simulink model "SF049A_LoaMgr"  (R2013b)
settings: Solver=FixedStepDiscrete  SolverMode=SingleTasking  StartTime=0.0  StopTime=1  FixedStep=0.002  RelTol=1e-3
values from neighbouring files (symbols this model uses):
  CURRMEASLOAMTGTNMASK_CNT_U08 = DataDict.Constant    [SF049A_LoaMgr_DataDict.m]
  IVTRLOAMTGTNMASK_CNT_U08 = DataDict.Constant    [SF049A_LoaMgr_DataDict.m]
  LOAMAXSLEW_ULSPERSEC_F32 = DataDict.Constant    [SF049A_LoaMgr_DataDict.m]
  LoaMgrCurrIvtrMtgtnRate = DataDict.Calibration    [SF049A_LoaMgr_DataDict.m]
  LoaMgrCurrIvtrMtgtnSca = DataDict.Calibration    [SF049A_LoaMgr_DataDict.m]
  LoaMgrCurrIvtrMtgtnScaZeroEna = DataDict.Calibration    [SF049A_LoaMgr_DataDict.m]
  LoaMgrCurrMeasIdptSig0Resp = DataDict.Calibration    [SF049A_LoaMgr_DataDict.m]
  LoaMgrCurrMeasIdptSig1Resp = DataDict.Calibration    [SF049A_LoaMgr_DataDict.m]
  LoaMgrCurrMeasIdptSig2Resp = DataDict.Calibration    [SF049A_LoaMgr_DataDict.m]
  LoaMgrCurrMeasIdptSigFltThd = DataDict.Calibration    [SF049A_LoaMgr_DataDict.m]
  LoaMgrCurrMeasMtgtnRate = DataDict.Calibration    [SF049A_LoaMgr_DataDict.m]
  LoaMgrCurrMeasMtgtnSca = DataDict.Calibration    [SF049A_LoaMgr_DataDict.m]
  LoaMgrCurrMeasMtgtnScaZeroEna = DataDict.Calibration    [SF049A_LoaMgr_DataDict.m]
  LoaMgrFadeOutStRate = DataDict.Calibration    [SF049A_LoaMgr_DataDict.m]
  LoaMgrHwTqIdptSig0NoTqLoaResp = DataDict.Calibration    [SF049A_LoaMgr_DataDict.m]
  LoaMgrHwTqIdptSig1NoTqLoaResp = DataDict.Calibration    [SF049A_LoaMgr_DataDict.m]
  LoaMgrHwTqIdptSig2Resp = DataDict.Calibration    [SF049A_LoaMgr_DataDict.m]
  LoaMgrHwTqIdptSig4Resp = DataDict.Calibration    [SF049A_LoaMgr_DataDict.m]
  LoaMgrHwTqIdptSigFltThd = DataDict.Calibration    [SF049A_LoaMgr_DataDict.m]
  LoaMgrHwTqLoaAvlResp = DataDict.Calibration    [SF049A_LoaMgr_DataDict.m]
  LoaMgrIvtrIdptSig0Resp = DataDict.Calibration    [SF049A_LoaMgr_DataDict.m]
  LoaMgrIvtrIdptSig1Resp = DataDict.Calibration    [SF049A_LoaMgr_DataDict.m]
  LoaMgrIvtrIdptSig2Resp = DataDict.Calibration    [SF049A_LoaMgr_DataDict.m]
  LoaMgrIvtrIdptSigFltThd = DataDict.Calibration    [SF049A_LoaMgr_DataDict.m]
  LoaMgrIvtrMtgtnRate = DataDict.Calibration    [SF049A_LoaMgr_DataDict.m]
  LoaMgrIvtrMtgtnSca = DataDict.Calibration    [SF049A_LoaMgr_DataDict.m]
  LoaMgrIvtrMtgtnScaZeroEna = DataDict.Calibration    [SF049A_LoaMgr_DataDict.m]
  LoaMgrLimdStRate = DataDict.Calibration    [SF049A_LoaMgr_DataDict.m]
  LoaMgrLimdStSca = DataDict.Calibration    [SF049A_LoaMgr_DataDict.m]
  LoaMgrMotAgAvlSnsrlsResp = DataDict.Calibration    [SF049A_LoaMgr_DataDict.m]
  LoaMgrMotAgIdptSig0NoSnsrlsResp = DataDict.Calibration    [SF049A_LoaMgr_DataDict.m]
  LoaMgrMotAgIdptSig1NoSnsrlsResp = DataDict.Calibration    [SF049A_LoaMgr_DataDict.m]
  LoaMgrMotAgIdptSig2Resp = DataDict.Calibration    [SF049A_LoaMgr_DataDict.m]
  LoaMgrMotAgIdptSig3Resp = DataDict.Calibration    [SF049A_LoaMgr_DataDict.m]
  LoaMgrMotAgIdptSigFltThd = DataDict.Calibration    [SF049A_LoaMgr_DataDict.m]
  LoaMgrMotAgMtgtnRate = DataDict.Calibration    [SF049A_LoaMgr_DataDict.m]
  LoaMgrMotAgMtgtnSca = DataDict.Calibration    [SF049A_LoaMgr_DataDict.m]
  LoaMgrMotAgMtgtnScaZeroEna = DataDict.Calibration    [SF049A_LoaMgr_DataDict.m]
  LOASCAONE_ULS_F32 = DataDict.Constant    [SF049A_LoaMgr_DataDict.m]
  LOASCAZERO_ULS_F32 = DataDict.Constant    [SF049A_LoaMgr_DataDict.m]
  LOASTIMDTSHTDWN_CNT_U08 = DataDict.Constant    [SF049A_LoaMgr_DataDict.m]
  LOASTNORM_CNT_U08 = DataDict.Constant    [SF049A_LoaMgr_DataDict.m]
  LOASTSWMTGTN_CNT_U08 = DataDict.Constant    [SF049A_LoaMgr_DataDict.m]
  MAXCURRMEASIDPTSIGALLWD_CNT_U08 = DataDict.Constant    [SF049A_LoaMgr_DataDict.m]
  MAXHWTQIDPTSIGALLWD_CNT_U08 = DataDict.Constant    [SF049A_LoaMgr_DataDict.m]
  MAXIVTRIDPTSIGALLWD_CNT_U08 = DataDict.Constant    [SF049A_LoaMgr_DataDict.m]
  MAXMOTAGMECLIDPTSIGALLWD_CNT_U08 = DataDict.Constant    [SF049A_LoaMgr_DataDict.m]
  NODEBSTEP_CNT_U16 = DataDict.Constant    [SF049A_LoaMgr_DataDict.m]
undefined symbols (not defined in the file or in its folder): LoaSt1, NtcNr1, NtcSts1, SigQlfr1
libraries: simulink x43, NxtrMin x4, NxtrMax x4, NxtrLim x2
(part 4 of 8)

== system SF049A_LoaMgr/LoaMgr/LoaMgrPer1/Arbitrate_Responses/SelFinalResp ==
  note: Pick the most severe of all the requested responses.
      |
      | 5 Immediate Shutdown  (most severe)
      | 4 Controlled Shutdown
      | 3 FadeOut
      | 2 Software-based Mitigation
      | 1 Reduced Performance
      | 0 Normal Operation       (least severe)
  MultiMtgtnResp : Inport  RequirementInfo="{'linktype_rmi_doors' '0000bab3 (/E-STEER Core/SubSystem Specifications/Application Functions/SF049A Loss of Assist Manager)' '#SF049A_84' 'true' 'REQ:  SF049A_84' '' } %GIDa_54734b91_5608_48ea_8068_35ba43353152"
  HwTqResp : Inport  RequirementInfo="{'linktype_rmi_doors' '0000bab3 (/E-STEER Core/SubSystem Specifications/Application Functions/SF049A Loss of Assist Manager)' '#SF049A_84' 'true' 'REQ:  SF049A_84' '' } %GIDa_c3761ef3_9e8d_4836_b42a_0c95799c1a90"  Port=2
  MotAgResp : Inport  RequirementInfo="{'linktype_rmi_doors' '0000bab3 (/E-STEER Core/SubSystem Specifications/Application Functions/SF049A Loss of Assist Manager)' '#SF049A_84' 'true' 'REQ:  SF049A_84' '' } %GIDa_49dd4887_96d7_4bb8_87d7_95367e2f50fb"  Port=3
  CurrMeasResp : Inport  RequirementInfo="{'linktype_rmi_doors' '0000bab3 (/E-STEER Core/SubSystem Specifications/Application Functions/SF049A Loss of Assist Manager)' '#SF049A_84' 'true' 'REQ:  SF049A_84' '' } %GIDa_84bf3833_e209_43be_a485_a63c89bdf184"  Port=4
  IvtrResp : Inport  RequirementInfo="{'linktype_rmi_doors' '0000bab3 (/E-STEER Core/SubSystem Specifications/Application Functions/SF049A Loss of Assist Manager)' '#SF049A_84' 'true' 'REQ:  SF049A_84' '' } %GIDa_dd1bf10a_41ed_4001_b74c_b927cf7e28c7"  Port=5
  CopyRight2 : Subsystem  Description=|  mask(Copyright Information){none=on}
      | Copyright info block.                                               
      |                                                                     
      | Place copyright information at the top of every subsystem in design.
      mask prompts: none "No parameters"
      mask help: Place copyright information at the top of every subsystem in design.
      mask Display:
      | NxtrConf = 'Nexteer Confidential';
      | 
      | sys = bdroot; %handle for the current model ("system")
      | first = get_param(sys,'Created');
      | first = first(end-3:end);  %year is last four digits
      | 
      | last = get_param(sys,'LastModifiedDate');
      | if isempty(last)
      |     last = datestr(now,'yyyy');
      | else
      |     last = last(end-3:end);
      | end
      | 
      | if strcmp(first,last)
      |     fprintf('%s -- Copyright %s Nexteer',NxtrConf,first)
      | else
      |     fprintf('%s -- %s%s- %s Nexteer',NxtrConf,char(169),first,last)
      | end
  F1 : Subsystem  RequirementInfo="{'linktype_rmi_doors' '0000bab3 (/E-STEER Core/SubSystem Specifications/Application Functions/SF049A Loss of Assist Manager)' '#SF049A_84' 'true' 'REQ:  SF049A_84' '' } %GIDa_43cd8944_2563_4272_8a81_50c14054d8ba"  TreatAsAtomicUnit=on
      settings: RTWSystemCode=Inline
  F2 : Subsystem  RequirementInfo="{'linktype_rmi_doors' '0000bab3 (/E-STEER Core/SubSystem Specifications/Application Functions/SF049A Loss of Assist Manager)' '#SF049A_84' 'true' 'REQ:  SF049A_84' '' } %GIDa_ad4154bc_5125_4599_b026_eafd9bdc2db0"  TreatAsAtomicUnit=on
      settings: RTWSystemCode=Inline
  Fade_Out : Subsystem  RequirementInfo="{'linktype_rmi_doors' '0000bab3 (/E-STEER Core/SubSystem Specifications/Application Functions/SF049A Loss of Assist Manager)' '#SF049A_84' 'true' 'REQ:  SF049A_84' '' } %GIDa_e73d73a9_eff4_41e2_9d30_bb96570f7ea9"  TreatAsAtomicUnit=on
      settings: RTWSystemCode=Inline
  Fade_Out1 : Subsystem  RequirementInfo="{'linktype_rmi_doors' '0000bab3 (/E-STEER Core/SubSystem Specifications/Application Functions/SF049A Loss of Assist Manager)' '#SF049A_84' 'true' 'REQ:  SF049A_84' '' } %GIDa_df16c958_8064_4140_9dc4_1de426c4fa71"  TreatAsAtomicUnit=on
      settings: RTWSystemCode=Inline
  Merge : Merge  RequirementInfo="{'linktype_rmi_doors' '0000bab3 (/E-STEER Core/SubSystem Specifications/Application Functions/SF049A Loss of Assist Manager)' '#SF049A_84' 'true' 'REQ:  SF049A_84' '' } %GIDa_bf53b07b_d7b9_4c96_87f9_e1354b1860d8"  Inputs=7
  MinMax : MinMax  RequirementInfo="{'linktype_rmi_doors' '0000bab3 (/E-STEER Core/SubSystem Specifications/Application Functions/SF049A Loss of Assist Manager)' '#SF049A_84' 'true' 'REQ:  SF049A_84' '' } %GIDa_e56cb4a9_e669_420e_96d1_e3295adf3ac5"  Function=max  Inputs=5
  Norm : Subsystem  RequirementInfo="{'linktype_rmi_doors' '0000bab3 (/E-STEER Core/SubSystem Specifications/Application Functions/SF049A Loss of Assist Manager)' '#SF049A_84' 'true' 'REQ:  SF049A_84' '' } %GIDa_79fd85a7_d991_4c90_8f93_f8588bbab999"  TreatAsAtomicUnit=on
      settings: RTWSystemCode=Inline
  Reduced : Subsystem  RequirementInfo="{'linktype_rmi_doors' '0000bab3 (/E-STEER Core/SubSystem Specifications/Application Functions/SF049A Loss of Assist Manager)' '#SF049A_84' 'true' 'REQ:  SF049A_84' '' } %GIDa_282ff44a_ee82_477d_994c_5b522cb9007f"  TreatAsAtomicUnit=on
      settings: RTWSystemCode=Inline
  SwBasd_Mtgtn : Subsystem  RequirementInfo="{'linktype_rmi_doors' '0000bab3 (/E-STEER Core/SubSystem Specifications/Application Functions/SF049A Loss of Assist Manager)' '#SF049A_84' 'true' 'REQ:  SF049A_84' '' } %GIDa_b7021016_4e5a_41fb_b8b0_41c73dc15fee"  TreatAsAtomicUnit=on
      settings: RTWSystemCode=Inline
  Switch Case : SwitchCase  RequirementInfo="{'linktype_rmi_doors' '0000bab3 (/E-STEER Core/SubSystem Specifications/Application Functions/SF049A Loss of Assist Manager)' '#SF049A_84' 'true' 'REQ:  SF049A_84' '' } %GIDa_44be8c31_fd6f_47a2_aa3d_457bbc5e3cf2"  CaseConditions={5,4,3,2,1,0}
  LoaSt : Outport  RequirementInfo="{'linktype_rmi_doors' '0000bab3 (/E-STEER Core/SubSystem Specifications/Application Functions/SF049A Loss of Assist Manager)' '#SF049A_84' 'true' 'REQ:  SF049A_84' '' } %GIDa_2917bb2b_4bd4_4079_ac09_4ef15e442a03"
  wires:
  SwBasd_Mtgtn/1(LoaSt) -> Merge/4
  Switch Case/7 -> Fade_Out1/Action
  MultiMtgtnResp/1 -> MinMax/1
  Fade_Out1/1(LoaSt) -> Merge/7
  Switch Case/6 -> Norm/Action
  Norm/1(LoaSt) -> Merge/6
  MinMax/1 -> Switch Case/1
  Switch Case/1 -> F1/Action
  F2/1(LoaSt) -> Merge/2
  Merge/1 -> LoaSt/1
  Fade_Out/1(LoaSt) -> Merge/3
  Switch Case/5 -> Reduced/Action
  Switch Case/3 -> Fade_Out/Action
  IvtrResp/1 -> MinMax/5
  Reduced/1(LoaSt) -> Merge/5
  Switch Case/2 -> F2/Action
  CurrMeasResp/1 -> MinMax/4
  F1/1(LoaSt) -> Merge/1
  HwTqResp/1 -> MinMax/2
  MotAgResp/1 -> MinMax/3
  Switch Case/4 -> SwBasd_Mtgtn/Action

== system SF049A_LoaMgr/LoaMgr/LoaMgrPer1/Assign_Scale/CopyRight2 ==

== system SF049A_LoaMgr/LoaMgr/LoaMgrPer1/Assign_Scale/F1 ==
  F1 : ActionPort  ActionType=else
  Constant1 : Constant  Value=LOASCAZERO_ULS_F32
  Constant2 : Constant  Value=LOAMAXSLEW_ULSPERSEC_F32
  CopyRight2 : Subsystem  Description=|  mask(Copyright Information){none=on}
      | Copyright info block.                                               
      |                                                                     
      | Place copyright information at the top of every subsystem in design.
      mask prompts: none "No parameters"
      mask help: Place copyright information at the top of every subsystem in design.
      mask Display:
      | NxtrConf = 'Nexteer Confidential';
      | 
      | sys = bdroot; %handle for the current model ("system")
      | first = get_param(sys,'Created');
      | first = first(end-3:end);  %year is last four digits
      | 
      | last = get_param(sys,'LastModifiedDate');
      | if isempty(last)
      |     last = datestr(now,'yyyy');
      | else
      |     last = last(end-3:end);
      | end
      | 
      | if strcmp(first,last)
      |     fprintf('%s -- Copyright %s Nexteer',NxtrConf,first)
      | else
      |     fprintf('%s -- %s%s- %s Nexteer',NxtrConf,char(169),first,last)
      | end
  Sca : Outport
  Rate : Outport  Port=2
  wires:
  Constant1/1 -> Sca/1
  Constant2/1 -> Rate/1

== system SF049A_LoaMgr/LoaMgr/LoaMgrPer1/Assign_Scale/F2 ==
  F2 : ActionPort  ActionType=elseif
  Constant1 : Constant  Value=LOASCAZERO_ULS_F32
  Constant2 : Constant  Value=LOAMAXSLEW_ULSPERSEC_F32
  CopyRight2 : Subsystem  Description=|  mask(Copyright Information){none=on}
      | Copyright info block.                                               
      |                                                                     
      | Place copyright information at the top of every subsystem in design.
      mask prompts: none "No parameters"
      mask help: Place copyright information at the top of every subsystem in design.
      mask Display:
      | NxtrConf = 'Nexteer Confidential';
      | 
      | sys = bdroot; %handle for the current model ("system")
      | first = get_param(sys,'Created');
      | first = first(end-3:end);  %year is last four digits
      | 
      | last = get_param(sys,'LastModifiedDate');
      | if isempty(last)
      |     last = datestr(now,'yyyy');
      | else
      |     last = last(end-3:end);
      | end
      | 
      | if strcmp(first,last)
      |     fprintf('%s -- Copyright %s Nexteer',NxtrConf,first)
      | else
      |     fprintf('%s -- %s%s- %s Nexteer',NxtrConf,char(169),first,last)
      | end
  Sca : Outport
  Rate : Outport  Port=2
  wires:
  Constant1/1 -> Sca/1
  Constant2/1 -> Rate/1

== system SF049A_LoaMgr/LoaMgr/LoaMgrPer1/Assign_Scale/Fade ==
  Fade : ActionPort  ActionType=elseif
  Constant1 : Constant  Value=LOASCAZERO_ULS_F32
  Constant2 : Constant  Value=LoaMgrFadeOutStRate
  CopyRight2 : Subsystem  Description=|  mask(Copyright Information){none=on}
      | Copyright info block.                                               
      |                                                                     
      | Place copyright information at the top of every subsystem in design.
      mask prompts: none "No parameters"
      mask help: Place copyright information at the top of every subsystem in design.
      mask Display:
      | NxtrConf = 'Nexteer Confidential';
      | 
      | sys = bdroot; %handle for the current model ("system")
      | first = get_param(sys,'Created');
      | first = first(end-3:end);  %year is last four digits
      | 
      | last = get_param(sys,'LastModifiedDate');
      | if isempty(last)
      |     last = datestr(now,'yyyy');
      | else
      |     last = last(end-3:end);
      | end
      | 
      | if strcmp(first,last)
      |     fprintf('%s -- Copyright %s Nexteer',NxtrConf,first)
      | else
      |     fprintf('%s -- %s%s- %s Nexteer',NxtrConf,char(169),first,last)
      | end
  Sca : Outport
  Rate : Outport  Port=2
  wires:
  Constant1/1 -> Sca/1
  Constant2/1 -> Rate/1

== system SF049A_LoaMgr/LoaMgr/LoaMgrPer1/Assign_Scale/Limd ==
  Reduced : ActionPort  ActionType=elseif
  Constant1 : Constant  Value=LoaMgrLimdStSca
  Constant2 : Constant  Value=LoaMgrLimdStRate
  CopyRight2 : Subsystem  Description=|  mask(Copyright Information){none=on}
      | Copyright info block.                                               
      |                                                                     
      | Place copyright information at the top of every subsystem in design.
      mask prompts: none "No parameters"
      mask help: Place copyright information at the top of every subsystem in design.
      mask Display:
      | NxtrConf = 'Nexteer Confidential';
      | 
      | sys = bdroot; %handle for the current model ("system")
      | first = get_param(sys,'Created');
      | first = first(end-3:end);  %year is last four digits
      | 
      | last = get_param(sys,'LastModifiedDate');
      | if isempty(last)
      |     last = datestr(now,'yyyy');
      | else
      |     last = last(end-3:end);
      | end
      | 
      | if strcmp(first,last)
      |     fprintf('%s -- Copyright %s Nexteer',NxtrConf,first)
      | else
      |     fprintf('%s -- %s%s- %s Nexteer',NxtrConf,char(169),first,last)
      | end
  Sca : Outport
  Rate : Outport  Port=2
  wires:
  Constant1/1 -> Sca/1
  Constant2/1 -> Rate/1

== system SF049A_LoaMgr/LoaMgr/LoaMgrPer1/Assign_Scale/Norm ==
  Normal : ActionPort  ActionType=then
  Constant1 : Constant  Value=LOASCAONE_ULS_F32
  Constant2 : Constant  Value=LOAMAXSLEW_ULSPERSEC_F32
  CopyRight2 : Subsystem  Description=|  mask(Copyright Information){none=on}
      | Copyright info block.                                               
      |                                                                     
      | Place copyright information at the top of every subsystem in design.
      mask prompts: none "No parameters"
      mask help: Place copyright information at the top of every subsystem in design.
      mask Display:
      | NxtrConf = 'Nexteer Confidential';
      | 
      | sys = bdroot; %handle for the current model ("system")
      | first = get_param(sys,'Created');
      | first = first(end-3:end);  %year is last four digits
      | 
      | last = get_param(sys,'LastModifiedDate');
      | if isempty(last)
      |     last = datestr(now,'yyyy');
      | else
      |     last = last(end-3:end);
      | end
      | 
      | if strcmp(first,last)
      |     fprintf('%s -- Copyright %s Nexteer',NxtrConf,first)
      | else
      |     fprintf('%s -- %s%s- %s Nexteer',NxtrConf,char(169),first,last)
      | end
  Sca : Outport
  Rate : Outport  Port=2
  wires:
  Constant1/1 -> Sca/1
  Constant2/1 -> Rate/1

== system SF049A_LoaMgr/LoaMgr/LoaMgrPer1/Assign_Scale/SwMtgtn ==
  SwMtgtnEn : Inport
  SwMtgtn : ActionPort  ActionType=elseif
  CopyRight2 : Subsystem  Description=|  mask(Copyright Information){none=on}
      | Copyright info block.                                               
      |                                                                     
      | Place copyright information at the top of every subsystem in design.
      mask prompts: none "No parameters"
      mask help: Place copyright information at the top of every subsystem in design.
      mask Display:
      | NxtrConf = 'Nexteer Confidential';
      | 
      | sys = bdroot; %handle for the current model ("system")
      | first = get_param(sys,'Created');
      | first = first(end-3:end);  %year is last four digits
      | 
      | last = get_param(sys,'LastModifiedDate');
      | if isempty(last)
      |     last = datestr(now,'yyyy');
      | else
      |     last = last(end-3:end);
      | end
      | 
      | if strcmp(first,last)
      |     fprintf('%s -- Copyright %s Nexteer',NxtrConf,first)
      | else
      |     fprintf('%s -- %s%s- %s Nexteer',NxtrConf,char(169),first,last)
      | end
  Data Store Read1 : DataStoreRead  Priority=1  DataStoreName=PrevVltgModSrc
  Data Store Read3 : DataStoreRead  Priority=1  DataStoreName=PrevMotAgLoaMtgtnEna
  Data Store Write1 : DataStoreWrite  Priority=2  DataStoreName=PrevVltgModSrc
  Data Store Write2 : DataStoreWrite  Priority=2  DataStoreName=PrevMotAgLoaMtgtnEna
  Demux : Demux
  HwTqTrue : Subsystem  RequirementInfo="{'linktype_rmi_doors' '0000bab3 (/E-STEER Core/SubSystem Specifications/Application Functions/SF049A Loss of Assist Manager)' '#SF049A_99' 'true' 'REQ:  SF049A_99' '' } %GIDa_7b14d0c5_f882_4af7_a11e_f83b181f5ec7"  TreatAsAtomicUnit=on
      settings: RTWSystemCode=Inline
  If : If  RequirementInfo="{'linktype_rmi_doors' '0000bab3 (/E-STEER Core/SubSystem Specifications/Application Functions/SF049A Loss of Assist Manager)' '#SF049A_99' 'true' 'REQ:  SF049A_99' '' ; 'linktype_rmi_doors' '0000bab3 (/E-STEER Core/SubSystem Specifications/Application Functions/SF049A Loss of Assist Manager)' '#SF049A_100' 'true' 'REQ:  SF049A_100' '' ; 'linktype_rmi_doors' '0000bab3 (/E-STEER Core/SubSystem Specifications/Application Functions/SF049A Loss of Assist Manager)' '#SF049A_107' 'true' 'REQ:  SF049A_107' '' ; 'linktype_rmi_doors' '0000bab3 (/E-STEER Core/SubSystem Specifications/Application Functions/SF049A Loss of Assist Manager)' '#SF049A_108' 'true' 'REQ:  SF049A_108' '' } %GIDa_e3d1a53d_44ce_4ebb_b524_70ede7db229d"  NumInputs=2  IfExpression=u1  ElseIfExpressions=u2
  MaskBooleans : Subsystem
  Merge : Merge  RequirementInfo="{'linktype_rmi_doors' '0000bab3 (/E-STEER Core/SubSystem Specifications/Application Functions/SF049A Loss of Assist Manager)' '#SF049A_99' 'true' 'REQ:  SF049A_99' '' ; 'linktype_rmi_doors' '0000bab3 (/E-STEER Core/SubSystem Specifications/Application Functions/SF049A Loss of Assist Manager)' '#SF049A_100' 'true' 'REQ:  SF049A_100' '' ; 'linktype_rmi_doors' '0000bab3 (/E-STEER Core/SubSystem Specifications/Application Functions/SF049A Loss of Assist Manager)' '#SF049A_107' 'true' 'REQ:  SF049A_107' '' ; 'linktype_rmi_doors' '0000bab3 (/E-STEER Core/SubSystem Specifications/Application Functions/SF049A Loss of Assist Manager)' '#SF049A_108' 'true' 'REQ:  SF049A_108' '' } %GIDa_35100d15_d4ea_4b72_b96f_d7a4004a9afa"  Inputs=3
  Merge1 : Merge  RequirementInfo="{'linktype_rmi_doors' '0000bab3 (/E-STEER Core/SubSystem Specifications/Application Functions/SF049A Loss of Assist Manager)' '#SF049A_99' 'true' 'REQ:  SF049A_99' '' ; 'linktype_rmi_doors' '0000bab3 (/E-STEER Core/SubSystem Specifications/Application Functions/SF049A Loss of Assist Manager)' '#SF049A_100' 'true' 'REQ:  SF049A_100' '' ; 'linktype_rmi_doors' '0000bab3 (/E-STEER Core/SubSystem Specifications/Application Functions/SF049A Loss of Assist Manager)' '#SF049A_107' 'true' 'REQ:  SF049A_107' '' ; 'linktype_rmi_doors' '0000bab3 (/E-STEER Core/SubSystem Specifications/Application Functions/SF049A Loss of Assist Manager)' '#SF049A_108' 'true' 'REQ:  SF049A_108' '' } %GIDa_747b6afd_1894_45a5_8818_39983e3267c2"  Inputs=3
  MotAgTrue : Subsystem  RequirementInfo="{'linktype_rmi_doors' '0000bab3 (/E-STEER Core/SubSystem Specifications/Application Functions/SF049A Loss of Assist Manager)' '#SF049A_100' 'true' 'REQ:  SF049A_100' '' } %GIDa_ffb79f06_004e_4cb8_9570_e4a0dcfed390"  TreatAsAtomicUnit=on
      settings: RTWSystemCode=Inline
  OthersTrue : Subsystem  RequirementInfo="{'linktype_rmi_doors' '0000bab3 (/E-STEER Core/SubSystem Specifications/Application Functions/SF049A Loss of Assist Manager)' '#SF049A_107' 'true' 'REQ:  SF049A_107' '' ; 'linktype_rmi_doors' '0000bab3 (/E-STEER Core/SubSystem Specifications/Application Functions/SF049A Loss of Assist Manager)' '#SF049A_108' 'true' 'REQ:  SF049A_108' '' } %GIDa_b6d2c039_d125_4c6d_9822_c6a7833ff1f7"  TreatAsAtomicUnit=on
      settings: RTWSystemCode=Inline
  Sca : Outport  RequirementInfo="{'linktype_rmi_doors' '0000bab3 (/E-STEER Core/SubSystem Specifications/Application Functions/SF049A Loss of Assist Manager)' '#SF049A_99' 'true' 'REQ:  SF049A_99' '' ; 'linktype_rmi_doors' '0000bab3 (/E-STEER Core/SubSystem Specifications/Application Functions/SF049A Loss of Assist Manager)' '#SF049A_100' 'true' 'REQ:  SF049A_100' '' ; 'linktype_rmi_doors' '0000bab3 (/E-STEER Core/SubSystem Specifications/Application Functions/SF049A Loss of Assist Manager)' '#SF049A_107' 'true' 'REQ:  SF049A_107' '' ; 'linktype_rmi_doors' '0000bab3 (/E-STEER Core/SubSystem Specifications/Application Functions/SF049A Loss of Assist Manager)' '#SF049A_108' 'true' 'REQ:  SF049A_108' '' } %GIDa_85f88b7e_b82d_4e96_8747_a438a2f288cc"
  Rate : Outport  RequirementInfo="{'linktype_rmi_doors' '0000bab3 (/E-STEER Core/SubSystem Specifications/Application Functions/SF049A Loss of Assist Manager)' '#SF049A_99' 'true' 'REQ:  SF049A_99' '' ; 'linktype_rmi_doors' '0000bab3 (/E-STEER Core/SubSystem Specifications/Application Functions/SF049A Loss of Assist Manager)' '#SF049A_100' 'true' 'REQ:  SF049A_100' '' ; 'linktype_rmi_doors' '0000bab3 (/E-STEER Core/SubSystem Specifications/Application Functions/SF049A Loss of Assist Manager)' '#SF049A_107' 'true' 'REQ:  SF049A_107' '' ; 'linktype_rmi_doors' '0000bab3 (/E-STEER Core/SubSystem Specifications/Application Functions/SF049A Loss of Assist Manager)' '#SF049A_108' 'true' 'REQ:  SF049A_108' '' } %GIDa_2e5e0cf3_0d2d_435e_bc0f_d301563c3972"  Port=2
  wires:
  SwMtgtnEn/1 -> Demux/1
  Demux/1 -> If/1  "HwTqLoaMtgtnEna"
  Demux/2 -> Data Store Write2/1, If/2  "MotAgLoaMtgtnEna"
  Demux/3 -> MaskBooleans/1(CurrMeasLoaMtgtnEna)  "CurrMeasLoaMtgtnEna"
  Demux/4 -> MaskBooleans/2(IvtrLoaMtgtnEna)  "IvtrLoaMtgtnEna"
  If/1 -> HwTqTrue/Action
  If/2 -> MotAgTrue/Action
  Data Store Read3/1 -> MotAgTrue/1(PrevMotAgLoaMtgtnEn)
  If/3 -> OthersTrue/Action
  MaskBooleans/1(VltgModSrc) -> OthersTrue/1(VltgModSrc), Data Store Write1/1
  Data Store Read1/1 -> OthersTrue/2(PrevVltgModSrc)
  HwTqTrue/1(Sca) -> Merge/1
  MotAgTrue/1(Sca) -> Merge/2
  HwTqTrue/2(Rate) -> Merge1/1
  MotAgTrue/2(Rate) -> Merge1/2
  OthersTrue/1(Sca) -> Merge/3
  OthersTrue/2(Rate) -> Merge1/3
  Merge/1 -> Sca/1
  Merge1/1 -> Rate/1

== system SF049A_LoaMgr/LoaMgr/LoaMgrPer1/Calc_Ivtr_State/CopyRight2 ==

== system SF049A_LoaMgr/LoaMgr/LoaMgrPer1/Calc_Ivtr_State/Ivtr1Sts_ELSE ==
  In1 : Inport
  Action Port : ActionPort  ActionType=else
  Out1 : Outport
  wires:
  In1/1 -> Out1/1

== system SF049A_LoaMgr/LoaMgr/LoaMgrPer1/Calc_Ivtr_State/Ivtr1Sts_THEN ==
  In1 : Inport
  Action Port : ActionPort  ActionType=then
  Out2 : Outport
  wires:
  In1/1 -> Out2/1

== system SF049A_LoaMgr/LoaMgr/LoaMgrPer1/Calc_Ivtr_State/Ivtr2Sts_ELSE ==
  In1 : Inport
  Action Port : ActionPort  ActionType=else
  Out1 : Outport
  wires:
  In1/1 -> Out1/1

== system SF049A_LoaMgr/LoaMgr/LoaMgrPer1/Calc_Ivtr_State/Ivtr2Sts_THEN ==
  In1 : Inport
  Action Port : ActionPort  ActionType=then
  Out1 : Outport
  wires:
  In1/1 -> Out1/1

== system SF049A_LoaMgr/LoaMgr/LoaMgrPer1/Latch_Inputs/CopyRight2 ==

== system SF049A_LoaMgr/LoaMgr/LoaMgrPer1/Latch_Inputs/RngLimCurrMeasIdptSig ==
  CurrMeasIdptSig : Inport  RequirementInfo="{'linktype_rmi_doors' '0000bab3 (/E-STEER Core/SubSystem Specifications/Application Functions/SF049A Loss of Assist Manager)' '#SF049A_188' 'true' 'REQ:  SF049A_188' '' } %GIDa_88563117_f185_42a9_91ba_188b17832b83"
  " 1" : Merge  RequirementInfo="{'linktype_rmi_doors' '0000bab3 (/E-STEER Core/SubSystem Specifications/Application Functions/SF049A Loss of Assist Manager)' '#SF049A_188' 'true' 'REQ:  SF049A_188' '' } %GIDa_993fa456_c567_4152_b9f7_8ff90298165c"
  Allw : Subsystem  RequirementInfo="{'linktype_rmi_doors' '0000bab3 (/E-STEER Core/SubSystem Specifications/Application Functions/SF049A Loss of Assist Manager)' '#SF049A_188' 'true' 'REQ:  SF049A_188' '' } %GIDa_364e1f96_9eca_433e_b74e_98ba966bab07"  TreatAsAtomicUnit=on
      settings: RTWSystemCode=Inline
  Compare To Constant1 : simulink/Logic and Bit Operations/Compare To Constant  RequirementInfo="{'linktype_rmi_doors' '0000bab3 (/E-STEER Core/SubSystem Specifications/Application Functions/SF049A Loss of Assist Manager)' '#SF049A_188' 'true' 'REQ:  SF049A_188' '' } %GIDa_f2549026_e3a3_4bd1_923b_13829a6545ca"  relop=>  const=MAXCURRMEASIDPTSIGALLWD_CNT_U08  OutDataTypeStr=boolean
  Constant2 : Constant  RequirementInfo="{'linktype_rmi_doors' '0000bab3 (/E-STEER Core/SubSystem Specifications/Application Functions/SF049A Loss of Assist Manager)' '#SF049A_188' 'true' 'REQ:  SF049A_188' '' } %GIDa_235f7593_bad0_4e34_b279_afe3238adad6"  Value=0  OutDataTypeStr=uint8
      settings: AttributesFormatString=%<OutDataTypeStr>
  CopyRight2 : Subsystem  Description=|  mask(Copyright Information){none=on}
      | Copyright info block.                                               
      |                                                                     
      | Place copyright information at the top of every subsystem in design.
      mask prompts: none "No parameters"
      mask help: Place copyright information at the top of every subsystem in design.
      mask Display:
      | NxtrConf = 'Nexteer Confidential';
      | 
      | sys = bdroot; %handle for the current model ("system")
      | first = get_param(sys,'Created');
      | first = first(end-3:end);  %year is last four digits
      | 
      | last = get_param(sys,'LastModifiedDate');
      | if isempty(last)
      |     last = datestr(now,'yyyy');
      | else
      |     last = last(end-3:end);
      | end
      | 
      | if strcmp(first,last)
      |     fprintf('%s -- Copyright %s Nexteer',NxtrConf,first)
      | else
      |     fprintf('%s -- %s%s- %s Nexteer',NxtrConf,char(169),first,last)
      | end
  DftVal : Subsystem  RequirementInfo="{'linktype_rmi_doors' '0000bab3 (/E-STEER Core/SubSystem Specifications/Application Functions/SF049A Loss of Assist Manager)' '#SF049A_188' 'true' 'REQ:  SF049A_188' '' } %GIDa_73a211b5_4341_4a34_ac97_9689c058f26e"  TreatAsAtomicUnit=on
      settings: RTWSystemCode=Inline
  Ivtr1Inactv_IF1 : If  RequirementInfo="{'linktype_rmi_doors' '0000bab3 (/E-STEER Core/SubSystem Specifications/Application Functions/SF049A Loss of Assist Manager)' '#SF049A_188' 'true' 'REQ:  SF049A_188' '' } %GIDa_4fbec484_a61e_4b48_82be_021e2ebd02aa"  IfExpression=u1
  RngLimdCurrMeasIdptSig : Outport  RequirementInfo="{'linktype_rmi_doors' '0000bab3 (/E-STEER Core/SubSystem Specifications/Application Functions/SF049A Loss of Assist Manager)' '#SF049A_188' 'true' 'REQ:  SF049A_188' '' } %GIDa_7209592e_646d_4505_afc1_842b5a6c0e86"
  wires:
  CurrMeasIdptSig/1 -> Allw/1(In1), Compare To Constant1/1
  Ivtr1Inactv_IF1/1 -> DftVal/Action
  Ivtr1Inactv_IF1/2 -> Allw/Action
  DftVal/1(Out2) -> " 1"/1
  " 1"/1 -> RngLimdCurrMeasIdptSig/1
  Constant2/1 -> DftVal/1(In1)
  Allw/1(Out1) -> " 1"/2
  Compare To Constant1/1 -> Ivtr1Inactv_IF1/1

== system SF049A_LoaMgr/LoaMgr/LoaMgrPer1/Latch_Inputs/RngLimHwTqIdptSig ==
  HwTqIdptSig : Inport  RequirementInfo="{'linktype_rmi_doors' '0000bab3 (/E-STEER Core/SubSystem Specifications/Application Functions/SF049A Loss of Assist Manager)' '#SF049A_186' 'true' 'REQ:  SF049A_186' '' } %GIDa_c7332a65_b89e_4090_b51e_6c587405479a"
  " 1" : Merge  RequirementInfo="{'linktype_rmi_doors' '0000bab3 (/E-STEER Core/SubSystem Specifications/Application Functions/SF049A Loss of Assist Manager)' '#SF049A_186' 'true' 'REQ:  SF049A_186' '' } %GIDa_997ca7c1_bda3_412d_b549_735c8cda0eed"
  Allw : Subsystem  RequirementInfo="{'linktype_rmi_doors' '0000bab3 (/E-STEER Core/SubSystem Specifications/Application Functions/SF049A Loss of Assist Manager)' '#SF049A_186' 'true' 'REQ:  SF049A_186' '' } %GIDa_dc6ae08f_e7f6_462f_8af1_036808ffc848"  TreatAsAtomicUnit=on
      settings: RTWSystemCode=Inline
  Compare To Constant1 : simulink/Logic and Bit Operations/Compare To Constant  RequirementInfo="{'linktype_rmi_doors' '0000bab3 (/E-STEER Core/SubSystem Specifications/Application Functions/SF049A Loss of Assist Manager)' '#SF049A_186' 'true' 'REQ:  SF049A_186' '' } %GIDa_1e850e0d_c0aa_464c_bf65_d68414a68e76"  relop=>  const=MAXHWTQIDPTSIGALLWD_CNT_U08  OutDataTypeStr=boolean
  Constant2 : Constant  RequirementInfo="{'linktype_rmi_doors' '0000bab3 (/E-STEER Core/SubSystem Specifications/Application Functions/SF049A Loss of Assist Manager)' '#SF049A_186' 'true' 'REQ:  SF049A_186' '' } %GIDa_2b00950e_a6a1_42cc_8845_cd23c0c37afb"  Value=0  OutDataTypeStr=uint8
      settings: AttributesFormatString=%<OutDataTypeStr>
  CopyRight2 : Subsystem  Description=|  mask(Copyright Information){none=on}
      | Copyright info block.                                               
      |                                                                     
      | Place copyright information at the top of every subsystem in design.
      mask prompts: none "No parameters"
      mask help: Place copyright information at the top of every subsystem in design.
      mask Display:
      | NxtrConf = 'Nexteer Confidential';
      | 
      | sys = bdroot; %handle for the current model ("system")
      | first = get_param(sys,'Created');
      | first = first(end-3:end);  %year is last four digits
      | 
      | last = get_param(sys,'LastModifiedDate');
      | if isempty(last)
      |     last = datestr(now,'yyyy');
      | else
      |     last = last(end-3:end);
      | end
      | 
      | if strcmp(first,last)
      |     fprintf('%s -- Copyright %s Nexteer',NxtrConf,first)
      | else
      |     fprintf('%s -- %s%s- %s Nexteer',NxtrConf,char(169),first,last)
      | end
  DftVal : Subsystem  RequirementInfo="{'linktype_rmi_doors' '0000bab3 (/E-STEER Core/SubSystem Specifications/Application Functions/SF049A Loss of Assist Manager)' '#SF049A_186' 'true' 'REQ:  SF049A_186' '' } %GIDa_8130d9f4_8675_49bb_ac84_ba41709e6ea0"  TreatAsAtomicUnit=on
      settings: RTWSystemCode=Inline
  Ivtr1Inactv_IF1 : If  RequirementInfo="{'linktype_rmi_doors' '0000bab3 (/E-STEER Core/SubSystem Specifications/Application Functions/SF049A Loss of Assist Manager)' '#SF049A_186' 'true' 'REQ:  SF049A_186' '' } %GIDa_cc914959_e899_4011_bab0_bef370f97e06"  IfExpression=u1
  RngLimdHwTqIdptSig : Outport  RequirementInfo="{'linktype_rmi_doors' '0000bab3 (/E-STEER Core/SubSystem Specifications/Application Functions/SF049A Loss of Assist Manager)' '#SF049A_186' 'true' 'REQ:  SF049A_186' '' } %GIDa_6b08fc90_0f14_4508_9276_a8af6d5d923b"
  wires:
  HwTqIdptSig/1 -> Allw/1(In1), Compare To Constant1/1
  Ivtr1Inactv_IF1/1 -> DftVal/Action
  Ivtr1Inactv_IF1/2 -> Allw/Action
  DftVal/1(Out2) -> " 1"/1
  " 1"/1 -> RngLimdHwTqIdptSig/1
  Constant2/1 -> DftVal/1(In1)
  Allw/1(Out1) -> " 1"/2
  Compare To Constant1/1 -> Ivtr1Inactv_IF1/1

== system SF049A_LoaMgr/LoaMgr/LoaMgrPer1/Latch_Inputs/RngLimMotAgMecIdptSig ==
  MotAgMeclIdptSig : Inport  RequirementInfo="{'linktype_rmi_doors' '0000bab3 (/E-STEER Core/SubSystem Specifications/Application Functions/SF049A Loss of Assist Manager)' '#SF049A_187' 'true' 'REQ:  SF049A_187' '' } %GIDa_ee979d2e_9731_4070_a924_d6094ed83dfb"
  " 1" : Merge  RequirementInfo="{'linktype_rmi_doors' '0000bab3 (/E-STEER Core/SubSystem Specifications/Application Functions/SF049A Loss of Assist Manager)' '#SF049A_187' 'true' 'REQ:  SF049A_187' '' } %GIDa_7af857e3_3071_4f93_b00e_cfb2f554b12a"
  Allw : Subsystem  RequirementInfo="{'linktype_rmi_doors' '0000bab3 (/E-STEER Core/SubSystem Specifications/Application Functions/SF049A Loss of Assist Manager)' '#SF049A_187' 'true' 'REQ:  SF049A_187' '' } %GIDa_7583d075_d8c6_49fd_8ebf_bb28e1febd36"  TreatAsAtomicUnit=on
      settings: RTWSystemCode=Inline
  Compare To Constant1 : simulink/Logic and Bit Operations/Compare To Constant  RequirementInfo="{'linktype_rmi_doors' '0000bab3 (/E-STEER Core/SubSystem Specifications/Application Functions/SF049A Loss of Assist Manager)' '#SF049A_187' 'true' 'REQ:  SF049A_187' '' } %GIDa_b4baf1eb_1525_483b_bc79_7d5f493a7d1b"  relop=>  const=MAXMOTAGMECLIDPTSIGALLWD_CNT_U08  OutDataTypeStr=boolean
  Constant2 : Constant  RequirementInfo="{'linktype_rmi_doors' '0000bab3 (/E-STEER Core/SubSystem Specifications/Application Functions/SF049A Loss of Assist Manager)' '#SF049A_187' 'true' 'REQ:  SF049A_187' '' } %GIDa_58d56a0b_a1b8_4aa3_b685_bfbc1819c890"  Value=0  OutDataTypeStr=uint8
      settings: AttributesFormatString=%<OutDataTypeStr>
  CopyRight2 : Subsystem  Description=|  mask(Copyright Information){none=on}
      | Copyright info block.                                               
      |                                                                     
      | Place copyright information at the top of every subsystem in design.
      mask prompts: none "No parameters"
      mask help: Place copyright information at the top of every subsystem in design.
      mask Display:
      | NxtrConf = 'Nexteer Confidential';
      | 
      | sys = bdroot; %handle for the current model ("system")
      | first = get_param(sys,'Created');
      | first = first(end-3:end);  %year is last four digits
      | 
      | last = get_param(sys,'LastModifiedDate');
      | if isempty(last)
      |     last = datestr(now,'yyyy');
      | else
      |     last = last(end-3:end);
      | end
      | 
      | if strcmp(first,last)
      |     fprintf('%s -- Copyright %s Nexteer',NxtrConf,first)
      | else
      |     fprintf('%s -- %s%s- %s Nexteer',NxtrConf,char(169),first,last)
      | end
  DftVal : Subsystem  RequirementInfo="{'linktype_rmi_doors' '0000bab3 (/E-STEER Core/SubSystem Specifications/Application Functions/SF049A Loss of Assist Manager)' '#SF049A_187' 'true' 'REQ:  SF049A_187' '' } %GIDa_055adde6_a232_4a35_a4c0_7c4f3cb2c4bf"  TreatAsAtomicUnit=on
      settings: RTWSystemCode=Inline
  Ivtr1Inactv_IF1 : If  RequirementInfo="{'linktype_rmi_doors' '0000bab3 (/E-STEER Core/SubSystem Specifications/Application Functions/SF049A Loss of Assist Manager)' '#SF049A_187' 'true' 'REQ:  SF049A_187' '' } %GIDa_56453199_a3fe_4e69_a9e4_42e51e23c7af"  IfExpression=u1
  RngLimdMotAgMecIdptSig : Outport  RequirementInfo="{'linktype_rmi_doors' '0000bab3 (/E-STEER Core/SubSystem Specifications/Application Functions/SF049A Loss of Assist Manager)' '#SF049A_187' 'true' 'REQ:  SF049A_187' '' } %GIDa_271aa4e2_383a_48be_96a5_342dca5c60e1"
  wires:
  Compare To Constant1/1 -> Ivtr1Inactv_IF1/1
  Allw/1(Out1) -> " 1"/2
  Constant2/1 -> DftVal/1(In1)
  " 1"/1 -> RngLimdMotAgMecIdptSig/1
  DftVal/1(Out2) -> " 1"/1
  Ivtr1Inactv_IF1/2 -> Allw/Action
  Ivtr1Inactv_IF1/1 -> DftVal/Action
  MotAgMeclIdptSig/1 -> Compare To Constant1/1, Allw/1(In1)

== system SF049A_LoaMgr/LoaMgr/LoaMgrPer1/Request_Responses/CopyRight1 ==

== system SF049A_LoaMgr/LoaMgr/LoaMgrPer1/Request_Responses/CurrMeasResp ==
  note: SWITCH CurrMeasIdptMin
      |     CASE 2
      |         CurrMeasResp = LoaMgrCurrMeasIdptSig2Resp
      |     CASE 1
      |          CurrMeasResp = LoaMgrCurrMeasIdptSig1Resp
      |     CASE ELSE
      |          CurrMeasResp = LoaMgrCurrMeasIdptSig0Resp
      | ENDSWITCH
  CurrMeasIdptMin : Inport  RequirementInfo="{'linktype_rmi_doors' '0000bab3 (/E-STEER Core/SubSystem Specifications/Application Functions/SF049A Loss of Assist Manager)' '#SF049A_64' 'true' 'REQ:  SF049A_64' '' } %GIDa_93860bc7_ac9a_4277_b7ce_bb00e281ac85"
  Constant : Constant  RequirementInfo="{'linktype_rmi_doors' '0000bab3 (/E-STEER Core/SubSystem Specifications/Application Functions/SF049A Loss of Assist Manager)' '#SF049A_64' 'true' 'REQ:  SF049A_64' '' } %GIDa_760fcdbc_8ae5_4ab2_85fb_b753151a90d0"  Value=LoaMgrCurrMeasIdptSig2Resp
  Constant1 : Constant  RequirementInfo="{'linktype_rmi_doors' '0000bab3 (/E-STEER Core/SubSystem Specifications/Application Functions/SF049A Loss of Assist Manager)' '#SF049A_64' 'true' 'REQ:  SF049A_64' '' } %GIDa_c4b4080a_c9e9_41ad_ac0e_a139bd416da4"  Value=LoaMgrCurrMeasIdptSig1Resp
  Constant2 : Constant  RequirementInfo="{'linktype_rmi_doors' '0000bab3 (/E-STEER Core/SubSystem Specifications/Application Functions/SF049A Loss of Assist Manager)' '#SF049A_64' 'true' 'REQ:  SF049A_64' '' } %GIDa_77dcd915_fe37_4786_8e65_88dc22b6161b"  Value=LoaMgrCurrMeasIdptSig0Resp
  CopyRight2 : Subsystem  Description=|  mask(Copyright Information){none=on}
      | Copyright info block.                                               
      |                                                                     
      | Place copyright information at the top of every subsystem in design.
      mask prompts: none "No parameters"
      mask help: Place copyright information at the top of every subsystem in design.
      mask Display:
      | NxtrConf = 'Nexteer Confidential';
      | 
      | sys = bdroot; %handle for the current model ("system")
      | first = get_param(sys,'Created');
      | first = first(end-3:end);  %year is last four digits
      | 
      | last = get_param(sys,'LastModifiedDate');
      | if isempty(last)
      |     last = datestr(now,'yyyy');
      | else
      |     last = last(end-3:end);
      | end
      | 
      | if strcmp(first,last)
      |     fprintf('%s -- Copyright %s Nexteer',NxtrConf,first)
      | else
      |     fprintf('%s -- %s%s- %s Nexteer',NxtrConf,char(169),first,last)
      | end
  Merge1 : Merge  RequirementInfo="{'linktype_rmi_doors' '0000bab3 (/E-STEER Core/SubSystem Specifications/Application Functions/SF049A Loss of Assist Manager)' '#SF049A_64' 'true' 'REQ:  SF049A_64' '' } %GIDa_b16e8e13_0fdb_439b_86f1_3a95249ed31a"  Inputs=3
  Switch Case : SwitchCase  RequirementInfo="{'linktype_rmi_doors' '0000bab3 (/E-STEER Core/SubSystem Specifications/Application Functions/SF049A Loss of Assist Manager)' '#SF049A_64' 'true' 'REQ:  SF049A_64' '' } %GIDa_407bfe53_3c47_4c35_85b2_cb2fe933bd5e"  CaseConditions={2,1}
  Two : Subsystem  RequirementInfo="{'linktype_rmi_doors' '0000bab3 (/E-STEER Core/SubSystem Specifications/Application Functions/SF049A Loss of Assist Manager)' '#SF049A_64' 'true' 'REQ:  SF049A_64' '' } %GIDa_c85f075a_7e92_4778_b78d_5faff8561f27"  TreatAsAtomicUnit=on
      settings: RTWSystemCode=Inline
  Zero_or_Invalid : Subsystem  RequirementInfo="{'linktype_rmi_doors' '0000bab3 (/E-STEER Core/SubSystem Specifications/Application Functions/SF049A Loss of Assist Manager)' '#SF049A_64' 'true' 'REQ:  SF049A_64' '' } %GIDa_b01904e9_1c77_4d62_b5c7_b3dde7d30158"  TreatAsAtomicUnit=on
      settings: RTWSystemCode=Inline
  one : Subsystem  RequirementInfo="{'linktype_rmi_doors' '0000bab3 (/E-STEER Core/SubSystem Specifications/Application Functions/SF049A Loss of Assist Manager)' '#SF049A_64' 'true' 'REQ:  SF049A_64' '' } %GIDa_9d3c4b7c_30c1_4793_ab77_cd957a13bbbe"  TreatAsAtomicUnit=on
      settings: RTWSystemCode=Inline
  CurrMeasResp : Outport  RequirementInfo="{'linktype_rmi_doors' '0000bab3 (/E-STEER Core/SubSystem Specifications/Application Functions/SF049A Loss of Assist Manager)' '#SF049A_64' 'true' 'REQ:  SF049A_64' '' } %GIDa_ebc48649_5b52_45f6_b24c_47c675a8c2cf"
  wires:
  CurrMeasIdptMin/1 -> Switch Case/1
  Switch Case/3 -> Zero_or_Invalid/Action
  Switch Case/1 -> Two/Action
  Constant/1 -> Two/1(Sig2Resp)
  Switch Case/2 -> one/Action
  Constant1/1 -> one/1(Sig1Resp)
  Two/1(CurrMeasResp) -> Merge1/1
  one/1(CurrMeasResp) -> Merge1/2
  Merge1/1 -> CurrMeasResp/1
  Zero_or_Invalid/1(CurrMeasResp) -> Merge1/3
  Constant2/1 -> Zero_or_Invalid/1(Sig0Resp)

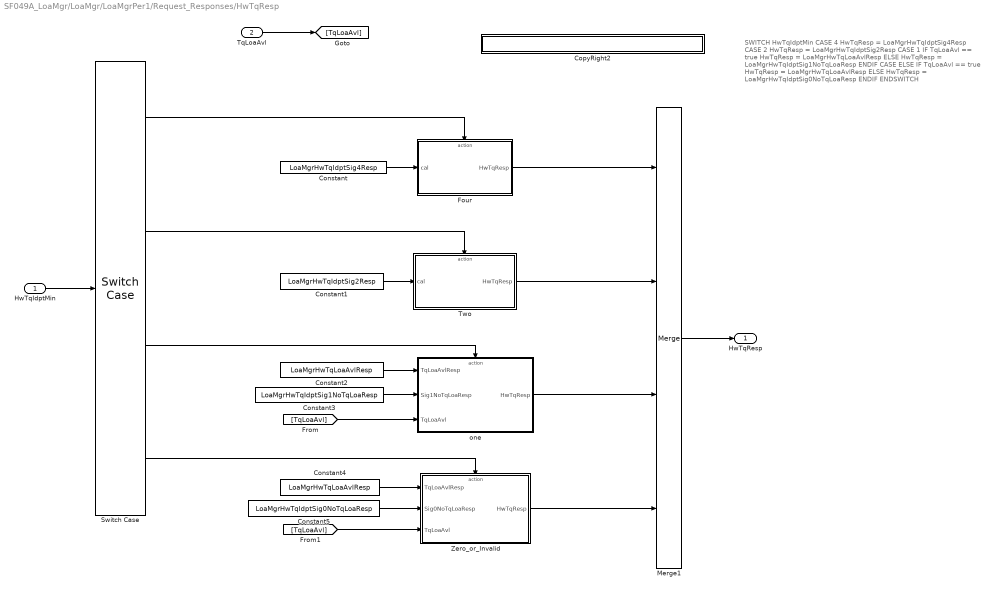
== system SF049A_LoaMgr/LoaMgr/LoaMgrPer1/Request_Responses/HwTqResp ==
  note: SWITCH HwTqIdptMin
      |     CASE 4
      |         HwTqResp = LoaMgrHwTqIdptSig4Resp
      |     CASE 2
      |         HwTqResp = LoaMgrHwTqIdptSig2Resp
      |     CASE 1
      |         IF TqLoaAvl == true
      |             HwTqResp = LoaMgrHwTqLoaAvlResp
      |         ELSE
      |             HwTqResp = LoaMgrHwTqIdptSig1NoTqLoaResp
      |         ENDIF
      |     CASE ELSE
      |         IF TqLoaAvl == true
      |             HwTqResp = LoaMgrHwTqLoaAvlResp
      |         ELSE
      |             HwTqResp = LoaMgrHwTqIdptSig0NoTqLoaResp
      |         ENDIF
      | ENDSWITCH
  HwTqIdptMin : Inport
  TqLoaAvl : Inport  Port=2
  Constant : Constant  RequirementInfo="{'linktype_rmi_doors' '0000bab3 (/E-STEER Core/SubSystem Specifications/Application Functions/SF049A Loss of Assist Manager)' '#SF049A_60' 'true' 'REQ:  SF049A_60' '' } %GIDa_01182c5d_dfae_4622_85c9_80cc03dd1594"  Value=LoaMgrHwTqIdptSig4Resp
  Constant1 : Constant  RequirementInfo="{'linktype_rmi_doors' '0000bab3 (/E-STEER Core/SubSystem Specifications/Application Functions/SF049A Loss of Assist Manager)' '#SF049A_60' 'true' 'REQ:  SF049A_60' '' } %GIDa_64629da8_2b7f_4ee3_aeb4_cf44a17abb13"  Value=LoaMgrHwTqIdptSig2Resp
  Constant2 : Constant  RequirementInfo="{'linktype_rmi_doors' '0000bab3 (/E-STEER Core/SubSystem Specifications/Application Functions/SF049A Loss of Assist Manager)' '#SF049A_60' 'true' 'REQ:  SF049A_60' '' } %GIDa_b33725aa_2356_4a5a_a648_b3fe8a2b91df"  Value=LoaMgrHwTqLoaAvlResp
  Constant3 : Constant  RequirementInfo="{'linktype_rmi_doors' '0000bab3 (/E-STEER Core/SubSystem Specifications/Application Functions/SF049A Loss of Assist Manager)' '#SF049A_60' 'true' 'REQ:  SF049A_60' '' } %GIDa_789f388f_cecb_4150_9c0c_b904434a1ad0"  Value=LoaMgrHwTqIdptSig1NoTqLoaResp
  Constant4 : Constant  RequirementInfo="{'linktype_rmi_doors' '0000bab3 (/E-STEER Core/SubSystem Specifications/Application Functions/SF049A Loss of Assist Manager)' '#SF049A_60' 'true' 'REQ:  SF049A_60' '' } %GIDa_ce5ce8f8_b489_4b61_988d_366c6f64cd33"  Value=LoaMgrHwTqLoaAvlResp
  Constant5 : Constant  RequirementInfo="{'linktype_rmi_doors' '0000bab3 (/E-STEER Core/SubSystem Specifications/Application Functions/SF049A Loss of Assist Manager)' '#SF049A_60' 'true' 'REQ:  SF049A_60' '' } %GIDa_a4a8ddaf_9241_4e09_9edb_8417600be61b"  Value=LoaMgrHwTqIdptSig0NoTqLoaResp
  CopyRight2 : Subsystem  Description=|  mask(Copyright Information){none=on}
      | Copyright info block.                                               
      |                                                                     
      | Place copyright information at the top of every subsystem in design.
      mask prompts: none "No parameters"
      mask help: Place copyright information at the top of every subsystem in design.
      mask Display:
      | NxtrConf = 'Nexteer Confidential';
      | 
      | sys = bdroot; %handle for the current model ("system")
      | first = get_param(sys,'Created');
      | first = first(end-3:end);  %year is last four digits
      | 
      | last = get_param(sys,'LastModifiedDate');
      | if isempty(last)
      |     last = datestr(now,'yyyy');
      | else
      |     last = last(end-3:end);
      | end
      | 
      | if strcmp(first,last)
      |     fprintf('%s -- Copyright %s Nexteer',NxtrConf,first)
      | else
      |     fprintf('%s -- %s%s- %s Nexteer',NxtrConf,char(169),first,last)
      | end
  Four : Subsystem  RequirementInfo="{'linktype_rmi_doors' '0000bab3 (/E-STEER Core/SubSystem Specifications/Application Functions/SF049A Loss of Assist Manager)' '#SF049A_60' 'true' 'REQ:  SF049A_60' '' } %GIDa_9d7fd188_2fd9_453c_8bf2_c4382b584827"  TreatAsAtomicUnit=on
      settings: RTWSystemCode=Inline
  Merge1 : Merge  RequirementInfo="{'linktype_rmi_doors' '0000bab3 (/E-STEER Core/SubSystem Specifications/Application Functions/SF049A Loss of Assist Manager)' '#SF049A_60' 'true' 'REQ:  SF049A_60' '' } %GIDa_cb9b0186_ca41_4aff_b6ef_bac5223b4f4b"  Inputs=4
  Switch Case : SwitchCase  RequirementInfo="{'linktype_rmi_doors' '0000bab3 (/E-STEER Core/SubSystem Specifications/Application Functions/SF049A Loss of Assist Manager)' '#SF049A_60' 'true' 'REQ:  SF049A_60' '' } %GIDa_0010a48e_3ed3_4983_81ce_d08e8f0cb1a0"  CaseConditions={4,2,1}
  Two : Subsystem  RequirementInfo="{'linktype_rmi_doors' '0000bab3 (/E-STEER Core/SubSystem Specifications/Application Functions/SF049A Loss of Assist Manager)' '#SF049A_60' 'true' 'REQ:  SF049A_60' '' } %GIDa_27cf6e94_220f_4666_aefd_d2a3a26bd174"  TreatAsAtomicUnit=on
      settings: RTWSystemCode=Inline
  Zero_or_Invalid : Subsystem  RequirementInfo="{'linktype_rmi_doors' '0000bab3 (/E-STEER Core/SubSystem Specifications/Application Functions/SF049A Loss of Assist Manager)' '#SF049A_60' 'true' 'REQ:  SF049A_60' '' } %GIDa_262eee4e_e374_4102_b81f_2ca45a5e66bc"  TreatAsAtomicUnit=on
      settings: RTWSystemCode=Inline
  one : Subsystem  RequirementInfo="{'linktype_rmi_doors' '0000bab3 (/E-STEER Core/SubSystem Specifications/Application Functions/SF049A Loss of Assist Manager)' '#SF049A_60' 'true' 'REQ:  SF049A_60' '' } %GIDa_e98a9488_7815_4428_a3f7_00adc3074c4d"  TreatAsAtomicUnit=on
      settings: RTWSystemCode=Inline
  HwTqResp : Outport  RequirementInfo="{'linktype_rmi_doors' '0000bab3 (/E-STEER Core/SubSystem Specifications/Application Functions/SF049A Loss of Assist Manager)' '#SF049A_60' 'true' 'REQ:  SF049A_60' '' } %GIDa_f8cfa34f_14c7_48af_a682_985a318c30dc"
  wires:
  Switch Case/3 -> one/Action
  HwTqIdptMin/1 -> Switch Case/1
  Switch Case/4 -> Zero_or_Invalid/Action
  Switch Case/1 -> Four/Action
  Constant/1 -> Four/1(cal)
  Switch Case/2 -> Two/Action
  Constant1/1 -> Two/1(cal)
  Constant2/1 -> one/1(TqLoaAvlResp)
  Constant3/1 -> one/2(Sig1NoTqLoaResp)
  TqLoaAvl/1 -> [TqLoaAvl]
  [TqLoaAvl] -> one/3(TqLoaAvl)
  Constant4/1 -> Zero_or_Invalid/1(TqLoaAvlResp)
  Constant5/1 -> Zero_or_Invalid/2(Sig0NoTqLoaResp)
  [TqLoaAvl] -> Zero_or_Invalid/3(TqLoaAvl)
  Four/1(HwTqResp) -> Merge1/1
  Two/1(HwTqResp) -> Merge1/2
  one/1(HwTqResp) -> Merge1/3
  Zero_or_Invalid/1(HwTqResp) -> Merge1/4
  Merge1/1 -> HwTqResp/1
